simulink model "PIL_position_controller_with_interfaces"  (R2023b)
settings: Solver=FixedStepAuto  StartTime=0.0  StopTime=10  RelTol=1e-5  EnableMultiTasking=on
undefined symbols (not defined in the file): DiscIntNeverNeededParam, K, Ts
libraries: simulink_extras x2, simulink x1
settings Model: CodeVerificationMode=processor-in-the-loop (pil)  ExtModeTrigDuration=10  Creator=paoli  LastModifiedBy=paoli
settings OptimizationCC: EnhancedBackFolding=on  PassReuseOutputArgsAs=Individual arguments  ZeroExternalMemoryAtStartup=off  ZeroInternalMemoryAtStartup=off  MaxStackSize=64  OptimizeBlockOrder=speed  DifferentSizesBufferReuse=on  OptimizationCustomize=off  EfficientTunableParamExpr=on
settings DebuggingCC: ParameterTunabilityLossMsg=error
settings HardwareCC: ProdBitPerPointer=32  ProdBitPerSizeT=32  ProdBitPerPtrDiffT=32  ProdLargestAtomicInteger=Long  ProdLargestAtomicFloat=Double  ProdWordSize=32  ProdLongLongMode=on  ProdHWDeviceType=ARM Compatible->ARM Cortex
settings SFSimCC: MATLABDynamicMemAlloc=off
settings RTWCC: Description=Embedded Coder  SystemTargetFile=ert.tlc  HardwareBoard=STM32 Nucleo F401RE  TemplateMakefile=ert_default_tmf  Toolchain=GNU Tools for ARM Embedded Processors  CodeExecutionProfiling=on  CodeProfilingInstrumentation=coarse
settings CodeAppCC: ForceParamTrailComments=on  IgnoreCustomStorageClasses=off  OperatorAnnotations=on  SimulinkDataObjDesc=on  SFDataObjDesc=on  InsertBlockDesc=on
settings ERTTargetCC: ExtModeTransport=3  ExtModeStaticAlloc=on  ExtModeStaticAllocSize=2000  ExtModeMexFile=ext_xcp  ExtModeIntrfLevel=Level2 - Open

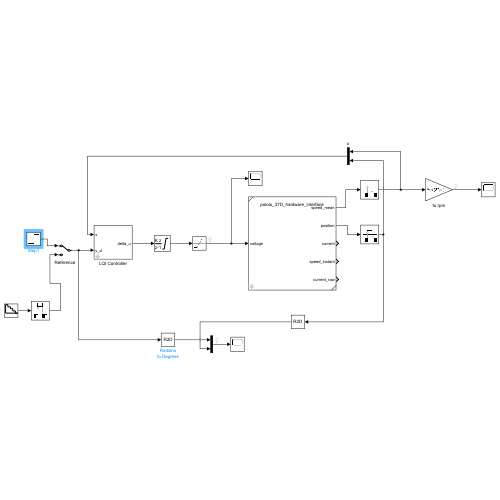
[thumbnail: Simulink's stored preview of the top-level diagram]
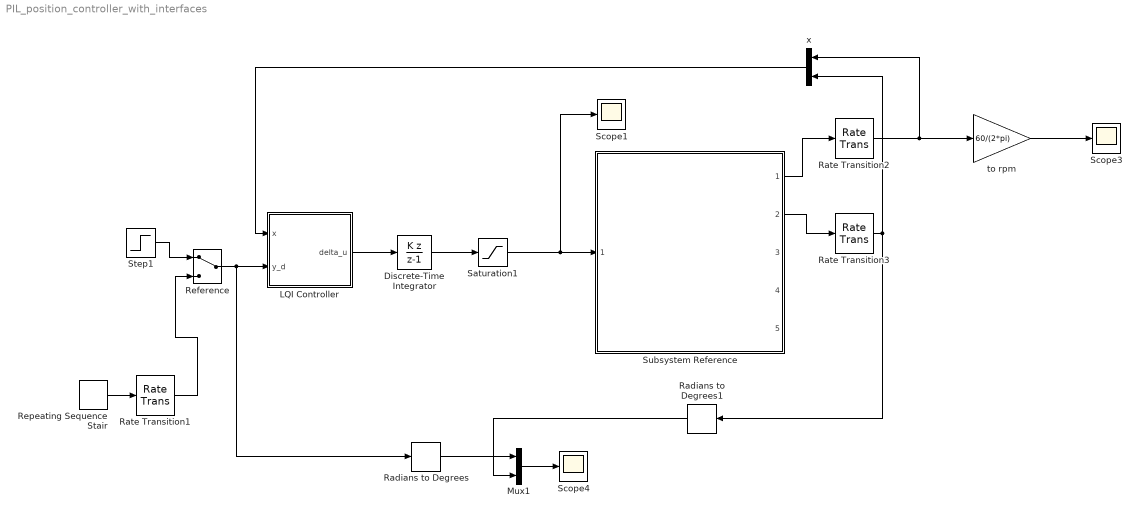
== system PIL_position_controller_with_interfaces ==
  Discrete-Time Integrator : DiscreteIntegrator  IntegratorMethod=Accumulation: Backward Euler  SampleTime=-1  LimitOutput=on  UpperSaturationLimit=12  LowerSaturationLimit=-12  ICPrevOutput=DiscIntNeverNeededParam  ICPrevScaledInput=DiscIntNeverNeededParam
  LQI Controller : Subsystem  mask{Ts=0.005}
  Mux1 : Mux  Inputs=2
  Radians to Degrees : simulink_extras/Transformations/Radians to Degrees
  Radians to Degrees1 : simulink_extras/Transformations/Radians to Degrees
  Rate Transition1 : RateTransition
  Rate Transition2 : RateTransition  OutPortSampleTime=Ts
  Rate Transition3 : RateTransition  OutPortSampleTime=Ts
  Reference : ManualSwitch
  Repeating Sequence Stair : simulink/Sources/Repeating Sequence Stair  OutValues=[0.160:-0.04:0].'  tsamp=2  OutMin=[]  OutMax=[]  OutDataTypeStr=double  OutputDataTypeScalingMode=double  OutDataType=fixdt(0,8)  ConRadixGroup=Best Precision: Vector-wise  OutScaling=2^-12
  Saturation1 : Saturate  UpperLimit=12  LowerLimit=-12
  Scope1 : Scope
  Scope3 : Scope
  Scope4 : Scope
  Step1 : Step  Time=0  After=pi  SampleTime=Ts
  Subsystem Reference : Subsystem  ReferencedSubsystem=pololu_37D_hardware_interface  Ts=Ts  pwmFreq=2000
  to rpm : Gain  Gain=60/(2*pi)
  x : Mux  Inputs=2
  wires:
  LQI Controller/1(delta_u) -> Discrete-Time Integrator/1
  Saturation1/1 -> Subsystem Reference/1, Scope1/1
  Reference/1 -> Radians to Degrees/1, LQI Controller/2(y_d)
  Discrete-Time Integrator/1 -> Saturation1/1
  Step1/1 -> Reference/1
  Repeating Sequence Stair/1 -> Rate Transition1/1
  Rate Transition1/1 -> Reference/2
  Subsystem Reference/1 -> Rate Transition2/1
  Subsystem Reference/2 -> Rate Transition3/1
  Rate Transition2/1 -> to rpm/1, x/1
  x/1 -> LQI Controller/1(x)
  Rate Transition3/1 -> x/2, Radians to Degrees1/1
  to rpm/1 -> Scope3/1
  Radians to Degrees1/1 -> Mux1/2
  Radians to Degrees/1 -> Mux1/1
  Mux1/1 -> Scope4/1

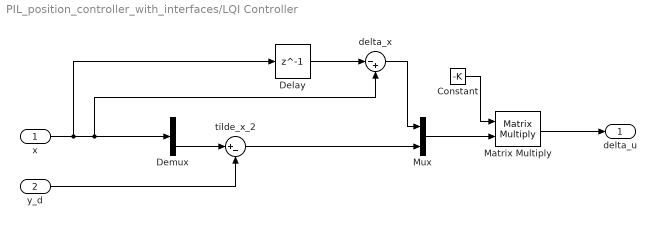
== system PIL_position_controller_with_interfaces/LQI Controller ==
  x : Inport  SampleTime=Ts
  y_d : Inport  Port=2  SampleTime=Ts
  Constant : Constant  Value=-K  VectorParams1D=off
  Delay : Delay  DelayLength=1  InitialCondition=[0;0]  SampleTime=Ts
  Demux : Demux  Outputs=2
  Matrix Multiply : Product  Multiplication=Matrix(*)
  Mux : Mux  Inputs=2
  delta_x : Sum  Inputs=|-+
  tilde_x_2 : Sum  Inputs=|+-
  delta_u : Outport  SampleTime=Ts
  wires:
  x/1 -> Delay/1, delta_x/2, Demux/1
  Mux/1 -> Matrix Multiply/2
  Demux/2 -> tilde_x_2/1
  y_d/1 -> tilde_x_2/2
  Delay/1 -> delta_x/1
  tilde_x_2/1 -> Mux/2
  Matrix Multiply/1 -> delta_u/1
  Constant/1 -> Matrix Multiply/1
  delta_x/1 -> Mux/1
